simulink model "W15_test_scenario_Map_cs"  (R2019a)
settings: Solver=FixedStepDiscrete  StartTime=0.0  StopTime=40  FixedStep=1/20  RelTol=1e-3
PreLoadFcn:
  | mbxruntime.callbacks.PreLoadFcn(bdroot);
  | check_NUTS_defined
  | model_closed = 0;
  | assignin('base',['model_closed_' bdroot],false);
PostLoadFcn:
  | mbxruntime.callbacks.PostLoadFcn(bdroot);
InitFcn:
  | mbxruntime.callbacks.InitFcn(bdroot);
StartFcn:
  | mbxruntime.callbacks.StartFcn(bdroot);
StopFcn:
  | mbxruntime.callbacks.StopFcn(bdroot);;
  | 
model workspace: external: MAT-File .\W15_test_scenario_Map_cs_hws.mat (data not in the file)
undefined symbols (not defined in the file or in its folder): DiscIntNeverNeededParam, Header, InitImageOutputDir, mbxruntime, Orientation, Poses, Poses_SL_Info, Position, tabledata, W15_test_scenario_Map_cs_169a523538b1c731, W15_test_scenario_Map_cs_214b7e80d33618ad, W15_test_scenario_Map_cs_2206180be8b5ba9f, W15_test_scenario_Map_cs_268dfee03830d0a5, W15_test_scenario_Map_cs_347647b3d0c1b5a3, W15_test_scenario_Map_cs_358fdd58312a0833, W15_test_scenario_Map_cs_5ba16ded7c4f6682, W15_test_scenario_Map_cs_615f57972979d30a, W15_test_scenario_Map_cs_62d25263d5c47c08, W15_test_scenario_Map_cs_6d9a3b1c984f4232, W15_test_scenario_Map_cs_8e30bed0320ac6d2, W15_test_scenario_Map_cs_91166841717f8002, W15_test_scenario_Map_cs_ab37b8bb7c840172, W15_test_scenario_Map_cs_Audi_A8_Sedan_1_Path_pathUniqueID, W15_test_scenario_Map_cs_bc72e7b61fa128bc, W15_test_scenario_Map_cs_Child_RegularAni_1_Path_pathUniqueID, W15_test_scenario_Map_cs_Child_RegularAni_2_Path_pathUniqueID, W15_test_scenario_Map_cs_e2220a37b0e8fe8c, W15_test_scenario_Map_cs_e86a0965b14e60bb, W15_test_scenario_Map_cs_Female_RegularAni_1_Path_pathUniqueID, W15_test_scenario_Map_cs_Male_RegularAni_1_Path_pathUniqueID, W15_test_scenario_Map_cs_Male_RegularAni_2_Path_pathUniqueID
libraries: simulink_extras x30, adeye_lib x14, simulink x10, robotlib x4, sharedtransform x2, PreScanSimulinkLibrary x2, PreScanUsefulBlocks x1
(part 4 of 8)

== system W15_test_scenario_Map_cs/STATE_Audi_A8_Sedan_1_bus ==
  STATE_Audi_A8_Sedan_1_bus : Inport  Tag=inport/StatePort  OutDataTypeStr=Bus: PRESCAN_STATEACTUATORDATA  PortDimensions=1  SampleTime=1/20  BusOutputAsStruct=on
  Actuator : S-Function  FunctionName=sfun_StateActuator  Parameters=mbxruntime.parameters.convert(UniqueID), mbxruntime.parameters.convert(TimeStep)  SFunctionDeploymentMode=off  EnableBusSupport=off  mask(PreScan Sink Block: State){UniqueID=18645, TimeStep=1/20}
      mask prompts: UniqueID "Auto-Assigned: Unique ID"; TimeStep "Auto-Assigned: Upload Period [s]"
      mask help:
      | The Actor State contains a vector signal of size (9x1), containing the following signals:
      |
      | -  Position    	(x,y,z)             	[m]
      | -  Velocity    	(vx,vy,vz)         	[m/s]
      | -  Angles       	(Roll, Pitch, Yaw)	[rad]
      |
      | The Actor state is defined in the global axis system.
      | The state is superponed on the Initial position defined in the GUI.
      |
      | For more information, please click Help.
      mask Help: eval('openHelp(222)')
      mask Display: image(imread('State.png'))
  wires:
  STATE_Audi_A8_Sedan_1_bus/1 -> Actuator/1

== system W15_test_scenario_Map_cs/STATE_BMW_X5_SUV_1_bus ==
  STATE_BMW_X5_SUV_1_bus : Inport  Tag=inport/StatePort  OutDataTypeStr=Bus: PRESCAN_STATEACTUATORDATA  PortDimensions=1  SampleTime=1/20  BusOutputAsStruct=on
  Actuator : S-Function  FunctionName=sfun_StateActuator  Parameters=mbxruntime.parameters.convert(UniqueID), mbxruntime.parameters.convert(TimeStep)  SFunctionDeploymentMode=off  EnableBusSupport=off  mask(PreScan Sink Block: State){UniqueID=9040, TimeStep=1/20}
      mask prompts: UniqueID "Auto-Assigned: Unique ID"; TimeStep "Auto-Assigned: Upload Period [s]"
      mask help:
      | The Actor State contains a vector signal of size (9x1), containing the following signals:
      |
      | -  Position    	(x,y,z)             	[m]
      | -  Velocity    	(vx,vy,vz)         	[m/s]
      | -  Angles       	(Roll, Pitch, Yaw)	[rad]
      |
      | The Actor state is defined in the global axis system.
      | The state is superponed on the Initial position defined in the GUI.
      |
      | For more information, please click Help.
      mask Help: eval('openHelp(222)')
      mask Display: image(imread('State.png'))
  wires:
  STATE_BMW_X5_SUV_1_bus/1 -> Actuator/1

== system W15_test_scenario_Map_cs/STATE_Child_RegularAni_1_bus ==
  STATE_Child_RegularAni_1_bus : Inport  Tag=inport/StatePort  OutDataTypeStr=Bus: PRESCAN_STATEACTUATORDATA  PortDimensions=1  SampleTime=1/20  BusOutputAsStruct=on
  Actuator : S-Function  FunctionName=sfun_StateActuator  Parameters=mbxruntime.parameters.convert(UniqueID), mbxruntime.parameters.convert(TimeStep)  SFunctionDeploymentMode=off  EnableBusSupport=off  mask(PreScan Sink Block: State){UniqueID=18395, TimeStep=1/20}
      mask prompts: UniqueID "Auto-Assigned: Unique ID"; TimeStep "Auto-Assigned: Upload Period [s]"
      mask help:
      | The Actor State contains a vector signal of size (9x1), containing the following signals:
      |
      | -  Position    	(x,y,z)             	[m]
      | -  Velocity    	(vx,vy,vz)         	[m/s]
      | -  Angles       	(Roll, Pitch, Yaw)	[rad]
      |
      | The Actor state is defined in the global axis system.
      | The state is superponed on the Initial position defined in the GUI.
      |
      | For more information, please click Help.
      mask Help: eval('openHelp(222)')
      mask Display: image(imread('State.png'))
  wires:
  STATE_Child_RegularAni_1_bus/1 -> Actuator/1

== system W15_test_scenario_Map_cs/STATE_Child_RegularAni_2_bus ==
  STATE_Child_RegularAni_2_bus : Inport  Tag=inport/StatePort  OutDataTypeStr=Bus: PRESCAN_STATEACTUATORDATA  PortDimensions=1  SampleTime=1/20  BusOutputAsStruct=on
  Actuator : S-Function  FunctionName=sfun_StateActuator  Parameters=mbxruntime.parameters.convert(UniqueID), mbxruntime.parameters.convert(TimeStep)  SFunctionDeploymentMode=off  EnableBusSupport=off  mask(PreScan Sink Block: State){UniqueID=18628, TimeStep=1/20}
      mask prompts: UniqueID "Auto-Assigned: Unique ID"; TimeStep "Auto-Assigned: Upload Period [s]"
      mask help:
      | The Actor State contains a vector signal of size (9x1), containing the following signals:
      |
      | -  Position    	(x,y,z)             	[m]
      | -  Velocity    	(vx,vy,vz)         	[m/s]
      | -  Angles       	(Roll, Pitch, Yaw)	[rad]
      |
      | The Actor state is defined in the global axis system.
      | The state is superponed on the Initial position defined in the GUI.
      |
      | For more information, please click Help.
      mask Help: eval('openHelp(222)')
      mask Display: image(imread('State.png'))
  wires:
  STATE_Child_RegularAni_2_bus/1 -> Actuator/1

== system W15_test_scenario_Map_cs/STATE_Citroen_C3_Hatchback_1_bus ==
  STATE_Citroen_C3_Hatchback_1_bus : Inport  Tag=inport/StatePort  OutDataTypeStr=Bus: PRESCAN_STATEACTUATORDATA  PortDimensions=1  SampleTime=1/20  BusOutputAsStruct=on
  Actuator : S-Function  FunctionName=sfun_StateActuator  Parameters=mbxruntime.parameters.convert(UniqueID), mbxruntime.parameters.convert(TimeStep)  SFunctionDeploymentMode=off  EnableBusSupport=off  mask(PreScan Sink Block: State){UniqueID=18857, TimeStep=1/20}
      mask prompts: UniqueID "Auto-Assigned: Unique ID"; TimeStep "Auto-Assigned: Upload Period [s]"
      mask help:
      | The Actor State contains a vector signal of size (9x1), containing the following signals:
      |
      | -  Position    	(x,y,z)             	[m]
      | -  Velocity    	(vx,vy,vz)         	[m/s]
      | -  Angles       	(Roll, Pitch, Yaw)	[rad]
      |
      | The Actor state is defined in the global axis system.
      | The state is superponed on the Initial position defined in the GUI.
      |
      | For more information, please click Help.
      mask Help: eval('openHelp(222)')
      mask Display: image(imread('State.png'))
  wires:
  STATE_Citroen_C3_Hatchback_1_bus/1 -> Actuator/1

== system W15_test_scenario_Map_cs/STATE_Female_RegularAni_1_bus ==
  STATE_Female_RegularAni_1_bus : Inport  Tag=inport/StatePort  OutDataTypeStr=Bus: PRESCAN_STATEACTUATORDATA  PortDimensions=1  SampleTime=1/20  BusOutputAsStruct=on
  Actuator : S-Function  FunctionName=sfun_StateActuator  Parameters=mbxruntime.parameters.convert(UniqueID), mbxruntime.parameters.convert(TimeStep)  SFunctionDeploymentMode=off  EnableBusSupport=off  mask(PreScan Sink Block: State){UniqueID=18631, TimeStep=1/20}
      mask prompts: UniqueID "Auto-Assigned: Unique ID"; TimeStep "Auto-Assigned: Upload Period [s]"
      mask help:
      | The Actor State contains a vector signal of size (9x1), containing the following signals:
      |
      | -  Position    	(x,y,z)             	[m]
      | -  Velocity    	(vx,vy,vz)         	[m/s]
      | -  Angles       	(Roll, Pitch, Yaw)	[rad]
      |
      | The Actor state is defined in the global axis system.
      | The state is superponed on the Initial position defined in the GUI.
      |
      | For more information, please click Help.
      mask Help: eval('openHelp(222)')
      mask Display: image(imread('State.png'))
  wires:
  STATE_Female_RegularAni_1_bus/1 -> Actuator/1

== system W15_test_scenario_Map_cs/STATE_Ford_Fiesta_Hatchback_1_bus ==
  STATE_Ford_Fiesta_Hatchback_1_bus : Inport  Tag=inport/StatePort  OutDataTypeStr=Bus: PRESCAN_STATEACTUATORDATA  PortDimensions=1  SampleTime=1/20  BusOutputAsStruct=on
  Actuator : S-Function  FunctionName=sfun_StateActuator  Parameters=mbxruntime.parameters.convert(UniqueID), mbxruntime.parameters.convert(TimeStep)  SFunctionDeploymentMode=off  EnableBusSupport=off  mask(PreScan Sink Block: State){UniqueID=4876, TimeStep=1/20}
      mask prompts: UniqueID "Auto-Assigned: Unique ID"; TimeStep "Auto-Assigned: Upload Period [s]"
      mask help:
      | The Actor State contains a vector signal of size (9x1), containing the following signals:
      |
      | -  Position    	(x,y,z)             	[m]
      | -  Velocity    	(vx,vy,vz)         	[m/s]
      | -  Angles       	(Roll, Pitch, Yaw)	[rad]
      |
      | The Actor state is defined in the global axis system.
      | The state is superponed on the Initial position defined in the GUI.
      |
      | For more information, please click Help.
      mask Help: eval('openHelp(222)')
      mask Display: image(imread('State.png'))
  wires:
  STATE_Ford_Fiesta_Hatchback_1_bus/1 -> Actuator/1

== system W15_test_scenario_Map_cs/STATE_Male_RegularAni_1_bus ==
  STATE_Male_RegularAni_1_bus : Inport  Tag=inport/StatePort  OutDataTypeStr=Bus: PRESCAN_STATEACTUATORDATA  PortDimensions=1  SampleTime=1/20  BusOutputAsStruct=on
  Actuator : S-Function  FunctionName=sfun_StateActuator  Parameters=mbxruntime.parameters.convert(UniqueID), mbxruntime.parameters.convert(TimeStep)  SFunctionDeploymentMode=off  EnableBusSupport=off  mask(PreScan Sink Block: State){UniqueID=18634, TimeStep=1/20}
      mask prompts: UniqueID "Auto-Assigned: Unique ID"; TimeStep "Auto-Assigned: Upload Period [s]"
      mask help:
      | The Actor State contains a vector signal of size (9x1), containing the following signals:
      |
      | -  Position    	(x,y,z)             	[m]
      | -  Velocity    	(vx,vy,vz)         	[m/s]
      | -  Angles       	(Roll, Pitch, Yaw)	[rad]
      |
      | The Actor state is defined in the global axis system.
      | The state is superponed on the Initial position defined in the GUI.
      |
      | For more information, please click Help.
      mask Help: eval('openHelp(222)')
      mask Display: image(imread('State.png'))
  wires:
  STATE_Male_RegularAni_1_bus/1 -> Actuator/1

== system W15_test_scenario_Map_cs/STATE_Male_RegularAni_2_bus ==
  STATE_Male_RegularAni_2_bus : Inport  Tag=inport/StatePort  OutDataTypeStr=Bus: PRESCAN_STATEACTUATORDATA  PortDimensions=1  SampleTime=1/20  BusOutputAsStruct=on
  Actuator : S-Function  FunctionName=sfun_StateActuator  Parameters=mbxruntime.parameters.convert(UniqueID), mbxruntime.parameters.convert(TimeStep)  SFunctionDeploymentMode=off  EnableBusSupport=off  mask(PreScan Sink Block: State){UniqueID=18853, TimeStep=1/20}
      mask prompts: UniqueID "Auto-Assigned: Unique ID"; TimeStep "Auto-Assigned: Upload Period [s]"
      mask help:
      | The Actor State contains a vector signal of size (9x1), containing the following signals:
      |
      | -  Position    	(x,y,z)             	[m]
      | -  Velocity    	(vx,vy,vz)         	[m/s]
      | -  Angles       	(Roll, Pitch, Yaw)	[rad]
      |
      | The Actor state is defined in the global axis system.
      | The state is superponed on the Initial position defined in the GUI.
      |
      | For more information, please click Help.
      mask Help: eval('openHelp(222)')
      mask Display: image(imread('State.png'))
  wires:
  STATE_Male_RegularAni_2_bus/1 -> Actuator/1

== system W15_test_scenario_Map_cs/ScenarioEngine ==
  Clock : Clock
  sfun_ScenarioEngine : S-Function  FunctionName=sfun_ScenarioEngine  Parameters=TimeStep  SFunctionDeploymentMode=off  EnableBusSupport=off
  wires:
  Clock/1 -> sfun_ScenarioEngine/1

== system W15_test_scenario_Map_cs/Synchronizer ==
  Bus Selector1 : BusSelector  OutputSignals=FederateStopped
  Stop Simulation : Stop
  sfun_Synchronizer : S-Function  FunctionName=sfun_Synchronizer  Parameters=SampleTime  SFunctionDeploymentMode=off  EnableBusSupport=off  mask(Legacy Function){SFunctionSpec=void prescan_synchronizer_outputFcn(void ** work1, PRESCAN_SYNCHRONIZEDATA y1[1]), SampleTime=TimeStep, ShowSpec=on}
      mask prompts: SampleTime "Sample time (-1 for inherited):"; ShowSpec "Display function specification"
      mask help:
      | This block allows you to call the legacy functions specified by the following Legacy Code Tool definition:
      | def.SFunctionName = 'sfun_Synchronizer';
      | def.OutputFcnSpec = 'void prescan_synchronizer_outputFcn(void ** work1, PRESCAN_TIMESTAMPDATA u1[1], PRESCAN_SYNCHRONIZEDATA y1[1])';
      | def.StartFcnSpec = 'void prescan_synchronizer_startFcn(void ** work1)';
      | def.TerminateFcnSpec = 'void prescan_synchronizer_terminateFcn(void ** work1)';
      | def.HeaderFiles = {'prescan_synchronizer_data.h'};
      | def.HostLibFiles = {'sensorinterfaced.lib'};
      | def.IncPaths = {'src', 'C:\prescandev\vislibrary\vis\..\pimp\include\sensors\InterfaceRTW'};
      | def.SrcPaths = {'src'};
      | def.LibPaths = {'C:\\prescandev\\vislibrary_build\lib'};
      | def.SampleTime = 'parameterized';
      | def.Options.language = 'C';
      mask Help: <p>This block was generated automatically by the Legacy Code Tool. For detailed help on this tool, call<a href="matlab:legacy_code('help')"> legacy_code('help')</a>.</p>
      mask Callback ShowSpec:
      | if strcmp(get_param(gcbh, 'ShowSpec'), 'on')
      |   set_param(gcbh, 'MaskDisplay', sprintf('fprintf(''%s'');', get_param(gcbh, 'SFunctionSpec')));
      | else
      |   set_param(gcbh, 'MaskDisplay', sprintf('fprintf(''%s'');', get_param(gcbh, 'FunctionName')));
      | end
      mask Display: fprintf('void prescan_synchronizer_outputFcn(void ** work1, PRESCAN_SYNCHRONIZEDATA y1[1])');
  wires:
  sfun_Synchronizer/1 -> Bus Selector1/1
  Bus Selector1/1 -> Stop Simulation/1  "<FederateStopped>"

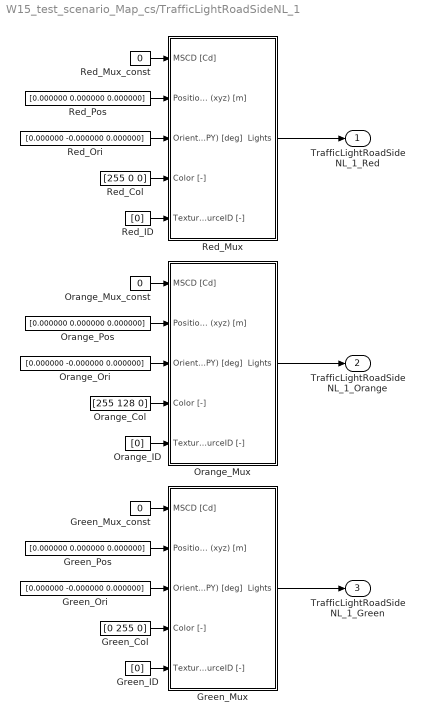
== system W15_test_scenario_Map_cs/TrafficLightRoadSideNL_1 ==
  Green_Col : Constant  Tag=VisuLightConst  Value=[0 255 0]
  Green_ID : Constant  Tag=VisuLightConst  Value=[0]
  Green_Mux : Subsystem  Tag=mux/ActiveLight  mask(PreScan User Interface: VisuActiveLight){}
      mask help:
      | The VisuActiveLight block provides a way for detailed animation of Light Sources, such as the indicator, brake, fog and main lights of a vehicle, or a light post.
      |
      | For more information, please click Help.
      settings: DeleteFcn=PreScanBlockDeleteFcn;
      mask Help: eval('openHelp(209)')
  Green_Mux_const : Constant  Tag=VisuLightConst  Value=0
  Green_Ori : Constant  Tag=VisuLightConst  Value=[0.000000 -0.000000 0.000000]
  Green_Pos : Constant  Tag=VisuLightConst  Value=[0.000000 0.000000 0.000000]
  Orange_Col : Constant  Tag=VisuLightConst  Value=[255 128 0]
  Orange_ID : Constant  Tag=VisuLightConst  Value=[0]
  Orange_Mux : Subsystem  Tag=mux/ActiveLight  mask(PreScan User Interface: VisuActiveLight){}
      mask help:
      | The VisuActiveLight block provides a way for detailed animation of Light Sources, such as the indicator, brake, fog and main lights of a vehicle, or a light post.
      |
      | For more information, please click Help.
      settings: DeleteFcn=PreScanBlockDeleteFcn;
      mask Help: eval('openHelp(209)')
  Orange_Mux_const : Constant  Tag=VisuLightConst  Value=0
  Orange_Ori : Constant  Tag=VisuLightConst  Value=[0.000000 -0.000000 0.000000]
  Orange_Pos : Constant  Tag=VisuLightConst  Value=[0.000000 0.000000 0.000000]
  Red_Col : Constant  Tag=VisuLightConst  Value=[255 0 0]
  Red_ID : Constant  Tag=VisuLightConst  Value=[0]
  Red_Mux : Subsystem  Tag=mux/ActiveLight  mask(PreScan User Interface: VisuActiveLight){}
      mask help:
      | The VisuActiveLight block provides a way for detailed animation of Light Sources, such as the indicator, brake, fog and main lights of a vehicle, or a light post.
      |
      | For more information, please click Help.
      settings: DeleteFcn=PreScanBlockDeleteFcn;
      mask Help: eval('openHelp(209)')
  Red_Mux_const : Constant  Tag=VisuLightConst  Value=0
  Red_Ori : Constant  Tag=VisuLightConst  Value=[0.000000 -0.000000 0.000000]
  Red_Pos : Constant  Tag=VisuLightConst  Value=[0.000000 0.000000 0.000000]
  TrafficLightRoadSideNL_1_Red : Outport  Tag=outport/Red  OutDataTypeStr=Bus: PRESCAN_VISULIGHTACTUATOR_DATA  SampleTime=1/20
  TrafficLightRoadSideNL_1_Orange : Outport  Tag=outport/Orange  Port=2  OutDataTypeStr=Bus: PRESCAN_VISULIGHTACTUATOR_DATA  SampleTime=1/20
  TrafficLightRoadSideNL_1_Green : Outport  Tag=outport/Green  Port=3  OutDataTypeStr=Bus: PRESCAN_VISULIGHTACTUATOR_DATA  SampleTime=1/20
  wires:
  Green_Mux_const/1 -> Green_Mux/1(MSCD [Cd])
  Orange_Mux_const/1 -> Orange_Mux/1(MSCD [Cd])
  Red_Mux_const/1 -> Red_Mux/1(MSCD [Cd])
  Red_Mux/1(Lights) -> TrafficLightRoadSideNL_1_Red/1
  Red_Pos/1 -> Red_Mux/2(Position (xyz) [m])
  Red_Ori/1 -> Red_Mux/3(Orientation (RPY) [deg])
  Red_Col/1 -> Red_Mux/4(Color [-])
  Red_ID/1 -> Red_Mux/5(TextureResourceID [-])
  Orange_Mux/1(Lights) -> TrafficLightRoadSideNL_1_Orange/1
  Orange_Pos/1 -> Orange_Mux/2(Position (xyz) [m])
  Orange_Ori/1 -> Orange_Mux/3(Orientation (RPY) [deg])
  Orange_Col/1 -> Orange_Mux/4(Color [-])
  Orange_ID/1 -> Orange_Mux/5(TextureResourceID [-])
  Green_Mux/1(Lights) -> TrafficLightRoadSideNL_1_Green/1
  Green_Pos/1 -> Green_Mux/2(Position (xyz) [m])
  Green_Ori/1 -> Green_Mux/3(Orientation (RPY) [deg])
  Green_Col/1 -> Green_Mux/4(Color [-])
  Green_ID/1 -> Green_Mux/5(TextureResourceID [-])

== system W15_test_scenario_Map_cs/TrafficLightRoadSideNL_1_Green ==
  TrafficLightRoadSideNL_1_Green : Inport  Tag=inport/Green  OutDataTypeStr=Bus: PRESCAN_VISULIGHTACTUATOR_DATA  SampleTime=1/20  BusOutputAsStruct=on
  Actuator : S-Function  FunctionName=sfun_VisuLightActuator  Parameters=mbxruntime.parameters.convert(UniqueID), mbxruntime.parameters.convert(LightName), mbxruntime.parameters.convert(PivotName), mbxruntime.parameters.convert(TextureResources), mbxruntime.parameters.convert(ColorsObjectName), mbxruntime.parameters.convert(MeshOnColor), mbxruntime.parameters.convert(MeshOffColor), tabledata, TimeStep  SFunctionDeploymentMode=off  EnableBusSupport=off  mask(PreScan Sink Block: VisuActiveLight){UniqueID=646, LightName=TrafficLightRoadSideNL_1.LightActuator_2_Green_ActiveLight, PivotName=TrafficLightRoadSideNL_1.Green, TextureResources={ 'Resources/LightMap/GeneralLight.png'}, ColorsObjectName=TrafficLightRoadSideNL_1.Green, MeshOnColor=[0  100    0  255    0  100    0  255  102  102  102  255    0  510    0  255], MeshOffColor=[0  100    0  255    0  100    0  255  102  102  102  255    0    0    0  255], TimeStep=1/20}
      mask prompts: UniqueID "Parent Unique Identifier"; LightName "Light"; PivotName "Pivot"; TextureResources "Texture Resources"; ColorsObjectName "Light Fixture Color Object"; MeshOnColor "Light Fixture On Color"; MeshOffColor "Light Fixture Off Color"; TimeStep "Simulink time step"
      mask help:
      | The VisuActiveLight block provides a way for detailed animation of Light Sources, such as the indicator, brake, fog and main lights of a vehicle, or a light post.
      |
      | For more information, please click Help.
      mask init:
      | [tabledata] = mbxruntime.parameters.table(UniqueID,LightName,PivotName,TextureResources,ColorsObjectName,MeshOnColor,MeshOffColor);
      mask Help: eval('openHelp(209)')
      mask Display: image(imread('HeadLight.png'))
  wires:
  TrafficLightRoadSideNL_1_Green/1 -> Actuator/1

== system W15_test_scenario_Map_cs/TrafficLightRoadSideNL_1_Orange ==
  TrafficLightRoadSideNL_1_Orange : Inport  Tag=inport/Orange  OutDataTypeStr=Bus: PRESCAN_VISULIGHTACTUATOR_DATA  SampleTime=1/20  BusOutputAsStruct=on
  Actuator : S-Function  FunctionName=sfun_VisuLightActuator  Parameters=mbxruntime.parameters.convert(UniqueID), mbxruntime.parameters.convert(LightName), mbxruntime.parameters.convert(PivotName), mbxruntime.parameters.convert(TextureResources), mbxruntime.parameters.convert(ColorsObjectName), mbxruntime.parameters.convert(MeshOnColor), mbxruntime.parameters.convert(MeshOffColor), tabledata, TimeStep  SFunctionDeploymentMode=off  EnableBusSupport=off  mask(PreScan Sink Block: VisuActiveLight){UniqueID=646, LightName=TrafficLightRoadSideNL_1.LightActuator_1_Orange_ActiveLight, PivotName=TrafficLightRoadSideNL_1.Orange, TextureResources={ 'Resources/LightMap/GeneralLight.png'}, ColorsObjectName=TrafficLightRoadSideNL_1.Orange, MeshOnColor=[100   50    0  255  100   50    0  255  102  102  102  255  510  256    0  255], MeshOffColor=[100   50    0  255  100   50    0  255  102  102  102  255    0    0    0  255], TimeStep=1/20}
      mask prompts: UniqueID "Parent Unique Identifier"; LightName "Light"; PivotName "Pivot"; TextureResources "Texture Resources"; ColorsObjectName "Light Fixture Color Object"; MeshOnColor "Light Fixture On Color"; MeshOffColor "Light Fixture Off Color"; TimeStep "Simulink time step"
      mask help:
      | The VisuActiveLight block provides a way for detailed animation of Light Sources, such as the indicator, brake, fog and main lights of a vehicle, or a light post.
      |
      | For more information, please click Help.
      mask init:
      | [tabledata] = mbxruntime.parameters.table(UniqueID,LightName,PivotName,TextureResources,ColorsObjectName,MeshOnColor,MeshOffColor);
      mask Help: eval('openHelp(209)')
      mask Display: image(imread('HeadLight.png'))
  wires:
  TrafficLightRoadSideNL_1_Orange/1 -> Actuator/1

== system W15_test_scenario_Map_cs/TrafficLightRoadSideNL_1_Red ==
  TrafficLightRoadSideNL_1_Red : Inport  Tag=inport/Red  OutDataTypeStr=Bus: PRESCAN_VISULIGHTACTUATOR_DATA  SampleTime=1/20  BusOutputAsStruct=on
  Actuator : S-Function  FunctionName=sfun_VisuLightActuator  Parameters=mbxruntime.parameters.convert(UniqueID), mbxruntime.parameters.convert(LightName), mbxruntime.parameters.convert(PivotName), mbxruntime.parameters.convert(TextureResources), mbxruntime.parameters.convert(ColorsObjectName), mbxruntime.parameters.convert(MeshOnColor), mbxruntime.parameters.convert(MeshOffColor), tabledata, TimeStep  SFunctionDeploymentMode=off  EnableBusSupport=off  mask(PreScan Sink Block: VisuActiveLight){UniqueID=646, LightName=TrafficLightRoadSideNL_1.LightActuator_0_Red_ActiveLight, PivotName=TrafficLightRoadSideNL_1.Red, TextureResources={ 'Resources/LightMap/GeneralLight.png'}, ColorsObjectName=TrafficLightRoadSideNL_1.Red, MeshOnColor=[100    0    0  255  100    0    0  255  102  102  102  255  510    0    0  255], MeshOffColor=[100    0    0  255  100    0    0  255  102  102  102  255    0    0    0  255], TimeStep=1/20}
      mask prompts: UniqueID "Parent Unique Identifier"; LightName "Light"; PivotName "Pivot"; TextureResources "Texture Resources"; ColorsObjectName "Light Fixture Color Object"; MeshOnColor "Light Fixture On Color"; MeshOffColor "Light Fixture Off Color"; TimeStep "Simulink time step"
      mask help:
      | The VisuActiveLight block provides a way for detailed animation of Light Sources, such as the indicator, brake, fog and main lights of a vehicle, or a light post.
      |
      | For more information, please click Help.
      mask init:
      | [tabledata] = mbxruntime.parameters.table(UniqueID,LightName,PivotName,TextureResources,ColorsObjectName,MeshOnColor,MeshOffColor);
      mask Help: eval('openHelp(209)')
      mask Display: image(imread('HeadLight.png'))
  wires:
  TrafficLightRoadSideNL_1_Red/1 -> Actuator/1

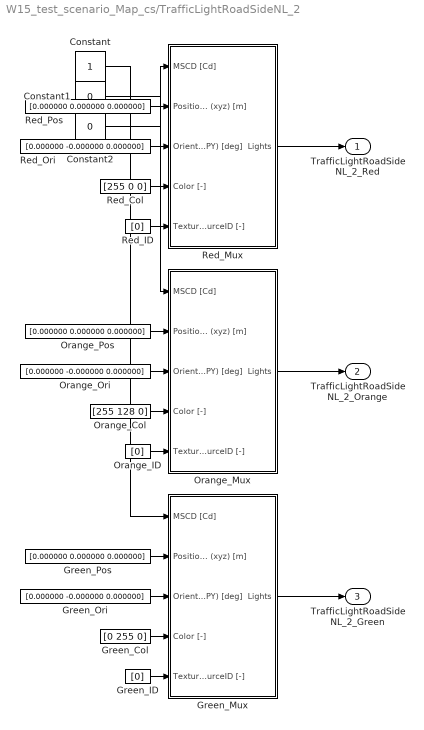
== system W15_test_scenario_Map_cs/TrafficLightRoadSideNL_2 ==
  Constant : Constant
  Constant1 : Constant  Value=0
  Constant2 : Constant  Value=0
  Green_Col : Constant  Tag=VisuLightConst  Value=[0 255 0]
  Green_ID : Constant  Tag=VisuLightConst  Value=[0]
  Green_Mux : Subsystem  Tag=mux/ActiveLight  mask(PreScan User Interface: VisuActiveLight){}
      mask help:
      | The VisuActiveLight block provides a way for detailed animation of Light Sources, such as the indicator, brake, fog and main lights of a vehicle, or a light post.
      |
      | For more information, please click Help.
      settings: DeleteFcn=PreScanBlockDeleteFcn;
      mask Help: eval('openHelp(209)')
  Green_Ori : Constant  Tag=VisuLightConst  Value=[0.000000 -0.000000 0.000000]
  Green_Pos : Constant  Tag=VisuLightConst  Value=[0.000000 0.000000 0.000000]
  Orange_Col : Constant  Tag=VisuLightConst  Value=[255 128 0]
  Orange_ID : Constant  Tag=VisuLightConst  Value=[0]
  Orange_Mux : Subsystem  Tag=mux/ActiveLight  mask(PreScan User Interface: VisuActiveLight){}
      mask help:
      | The VisuActiveLight block provides a way for detailed animation of Light Sources, such as the indicator, brake, fog and main lights of a vehicle, or a light post.
      |
      | For more information, please click Help.
      settings: DeleteFcn=PreScanBlockDeleteFcn;
      mask Help: eval('openHelp(209)')
  Orange_Ori : Constant  Tag=VisuLightConst  Value=[0.000000 -0.000000 0.000000]
  Orange_Pos : Constant  Tag=VisuLightConst  Value=[0.000000 0.000000 0.000000]
  Red_Col : Constant  Tag=VisuLightConst  Value=[255 0 0]
  Red_ID : Constant  Tag=VisuLightConst  Value=[0]
  Red_Mux : Subsystem  Tag=mux/ActiveLight  mask(PreScan User Interface: VisuActiveLight){}
      mask help:
      | The VisuActiveLight block provides a way for detailed animation of Light Sources, such as the indicator, brake, fog and main lights of a vehicle, or a light post.
      |
      | For more information, please click Help.
      settings: DeleteFcn=PreScanBlockDeleteFcn;
      mask Help: eval('openHelp(209)')
  Red_Ori : Constant  Tag=VisuLightConst  Value=[0.000000 -0.000000 0.000000]
  Red_Pos : Constant  Tag=VisuLightConst  Value=[0.000000 0.000000 0.000000]
  TrafficLightRoadSideNL_2_Red : Outport  Tag=outport/Red  OutDataTypeStr=Bus: PRESCAN_VISULIGHTACTUATOR_DATA  SampleTime=1/20
  TrafficLightRoadSideNL_2_Orange : Outport  Tag=outport/Orange  Port=2  OutDataTypeStr=Bus: PRESCAN_VISULIGHTACTUATOR_DATA  SampleTime=1/20
  TrafficLightRoadSideNL_2_Green : Outport  Tag=outport/Green  Port=3  OutDataTypeStr=Bus: PRESCAN_VISULIGHTACTUATOR_DATA  SampleTime=1/20
  wires:
  Constant/1 -> Green_Mux/1(MSCD [Cd])
  Constant1/1 -> Orange_Mux/1(MSCD [Cd])
  Constant2/1 -> Red_Mux/1(MSCD [Cd])
  Red_Mux/1(Lights) -> TrafficLightRoadSideNL_2_Red/1
  Red_Pos/1 -> Red_Mux/2(Position (xyz) [m])
  Red_Ori/1 -> Red_Mux/3(Orientation (RPY) [deg])
  Red_Col/1 -> Red_Mux/4(Color [-])
  Red_ID/1 -> Red_Mux/5(TextureResourceID [-])
  Orange_Mux/1(Lights) -> TrafficLightRoadSideNL_2_Orange/1
  Orange_Pos/1 -> Orange_Mux/2(Position (xyz) [m])
  Orange_Ori/1 -> Orange_Mux/3(Orientation (RPY) [deg])
  Orange_Col/1 -> Orange_Mux/4(Color [-])
  Orange_ID/1 -> Orange_Mux/5(TextureResourceID [-])
  Green_Mux/1(Lights) -> TrafficLightRoadSideNL_2_Green/1
  Green_Pos/1 -> Green_Mux/2(Position (xyz) [m])
  Green_Ori/1 -> Green_Mux/3(Orientation (RPY) [deg])
  Green_Col/1 -> Green_Mux/4(Color [-])
  Green_ID/1 -> Green_Mux/5(TextureResourceID [-])

== system W15_test_scenario_Map_cs/TrafficLightRoadSideNL_2_Green ==
  TrafficLightRoadSideNL_2_Green : Inport  Tag=inport/Green  OutDataTypeStr=Bus: PRESCAN_VISULIGHTACTUATOR_DATA  SampleTime=1/20  BusOutputAsStruct=on
  Actuator : S-Function  FunctionName=sfun_VisuLightActuator  Parameters=mbxruntime.parameters.convert(UniqueID), mbxruntime.parameters.convert(LightName), mbxruntime.parameters.convert(PivotName), mbxruntime.parameters.convert(TextureResources), mbxruntime.parameters.convert(ColorsObjectName), mbxruntime.parameters.convert(MeshOnColor), mbxruntime.parameters.convert(MeshOffColor), tabledata, TimeStep  SFunctionDeploymentMode=off  EnableBusSupport=off  mask(PreScan Sink Block: VisuActiveLight){UniqueID=647, LightName=TrafficLightRoadSideNL_2.LightActuator_2_Green_ActiveLight, PivotName=TrafficLightRoadSideNL_2.Green, TextureResources={ 'Resources/LightMap/GeneralLight.png'}, ColorsObjectName=TrafficLightRoadSideNL_2.Green, MeshOnColor=[0  100    0  255    0  100    0  255  102  102  102  255    0  510    0  255], MeshOffColor=[0  100    0  255    0  100    0  255  102  102  102  255    0    0    0  255], TimeStep=1/20}
      mask prompts: UniqueID "Parent Unique Identifier"; LightName "Light"; PivotName "Pivot"; TextureResources "Texture Resources"; ColorsObjectName "Light Fixture Color Object"; MeshOnColor "Light Fixture On Color"; MeshOffColor "Light Fixture Off Color"; TimeStep "Simulink time step"
      mask help:
      | The VisuActiveLight block provides a way for detailed animation of Light Sources, such as the indicator, brake, fog and main lights of a vehicle, or a light post.
      |
      | For more information, please click Help.
      mask init:
      | [tabledata] = mbxruntime.parameters.table(UniqueID,LightName,PivotName,TextureResources,ColorsObjectName,MeshOnColor,MeshOffColor);
      mask Help: eval('openHelp(209)')
      mask Display: image(imread('HeadLight.png'))
  wires:
  TrafficLightRoadSideNL_2_Green/1 -> Actuator/1

== system W15_test_scenario_Map_cs/TrafficLightRoadSideNL_2_Orange ==
  TrafficLightRoadSideNL_2_Orange : Inport  Tag=inport/Orange  OutDataTypeStr=Bus: PRESCAN_VISULIGHTACTUATOR_DATA  SampleTime=1/20  BusOutputAsStruct=on
  Actuator : S-Function  FunctionName=sfun_VisuLightActuator  Parameters=mbxruntime.parameters.convert(UniqueID), mbxruntime.parameters.convert(LightName), mbxruntime.parameters.convert(PivotName), mbxruntime.parameters.convert(TextureResources), mbxruntime.parameters.convert(ColorsObjectName), mbxruntime.parameters.convert(MeshOnColor), mbxruntime.parameters.convert(MeshOffColor), tabledata, TimeStep  SFunctionDeploymentMode=off  EnableBusSupport=off  mask(PreScan Sink Block: VisuActiveLight){UniqueID=647, LightName=TrafficLightRoadSideNL_2.LightActuator_1_Orange_ActiveLight, PivotName=TrafficLightRoadSideNL_2.Orange, TextureResources={ 'Resources/LightMap/GeneralLight.png'}, ColorsObjectName=TrafficLightRoadSideNL_2.Orange, MeshOnColor=[100   50    0  255  100   50    0  255  102  102  102  255  510  256    0  255], MeshOffColor=[100   50    0  255  100   50    0  255  102  102  102  255    0    0    0  255], TimeStep=1/20}
      mask prompts: UniqueID "Parent Unique Identifier"; LightName "Light"; PivotName "Pivot"; TextureResources "Texture Resources"; ColorsObjectName "Light Fixture Color Object"; MeshOnColor "Light Fixture On Color"; MeshOffColor "Light Fixture Off Color"; TimeStep "Simulink time step"
      mask help:
      | The VisuActiveLight block provides a way for detailed animation of Light Sources, such as the indicator, brake, fog and main lights of a vehicle, or a light post.
      |
      | For more information, please click Help.
      mask init:
      | [tabledata] = mbxruntime.parameters.table(UniqueID,LightName,PivotName,TextureResources,ColorsObjectName,MeshOnColor,MeshOffColor);
      mask Help: eval('openHelp(209)')
      mask Display: image(imread('HeadLight.png'))
  wires:
  TrafficLightRoadSideNL_2_Orange/1 -> Actuator/1

== system W15_test_scenario_Map_cs/TrafficLightRoadSideNL_2_Red ==
  TrafficLightRoadSideNL_2_Red : Inport  Tag=inport/Red  OutDataTypeStr=Bus: PRESCAN_VISULIGHTACTUATOR_DATA  SampleTime=1/20  BusOutputAsStruct=on
  Actuator : S-Function  FunctionName=sfun_VisuLightActuator  Parameters=mbxruntime.parameters.convert(UniqueID), mbxruntime.parameters.convert(LightName), mbxruntime.parameters.convert(PivotName), mbxruntime.parameters.convert(TextureResources), mbxruntime.parameters.convert(ColorsObjectName), mbxruntime.parameters.convert(MeshOnColor), mbxruntime.parameters.convert(MeshOffColor), tabledata, TimeStep  SFunctionDeploymentMode=off  EnableBusSupport=off  mask(PreScan Sink Block: VisuActiveLight){UniqueID=647, LightName=TrafficLightRoadSideNL_2.LightActuator_0_Red_ActiveLight, PivotName=TrafficLightRoadSideNL_2.Red, TextureResources={ 'Resources/LightMap/GeneralLight.png'}, ColorsObjectName=TrafficLightRoadSideNL_2.Red, MeshOnColor=[100    0    0  255  100    0    0  255  102  102  102  255  510    0    0  255], MeshOffColor=[100    0    0  255  100    0    0  255  102  102  102  255    0    0    0  255], TimeStep=1/20}
      mask prompts: UniqueID "Parent Unique Identifier"; LightName "Light"; PivotName "Pivot"; TextureResources "Texture Resources"; ColorsObjectName "Light Fixture Color Object"; MeshOnColor "Light Fixture On Color"; MeshOffColor "Light Fixture Off Color"; TimeStep "Simulink time step"
      mask help:
      | The VisuActiveLight block provides a way for detailed animation of Light Sources, such as the indicator, brake, fog and main lights of a vehicle, or a light post.
      |
      | For more information, please click Help.
      mask init:
      | [tabledata] = mbxruntime.parameters.table(UniqueID,LightName,PivotName,TextureResources,ColorsObjectName,MeshOnColor,MeshOffColor);
      mask Help: eval('openHelp(209)')
      mask Display: image(imread('HeadLight.png'))
  wires:
  TrafficLightRoadSideNL_2_Red/1 -> Actuator/1

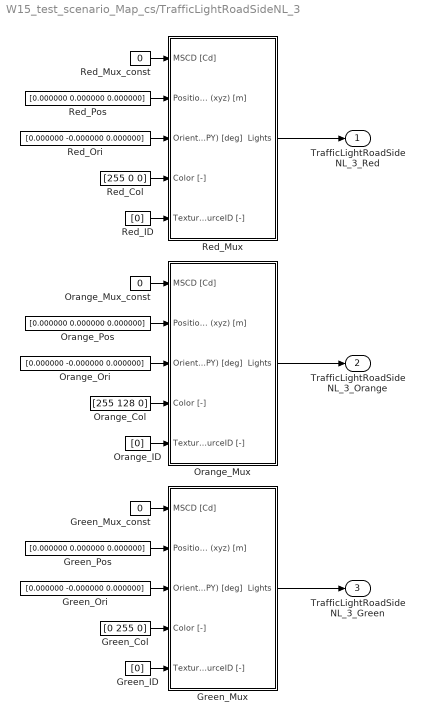
== system W15_test_scenario_Map_cs/TrafficLightRoadSideNL_3 ==
  Green_Col : Constant  Tag=VisuLightConst  Value=[0 255 0]
  Green_ID : Constant  Tag=VisuLightConst  Value=[0]
  Green_Mux : Subsystem  Tag=mux/ActiveLight  mask(PreScan User Interface: VisuActiveLight){}
      mask help:
      | The VisuActiveLight block provides a way for detailed animation of Light Sources, such as the indicator, brake, fog and main lights of a vehicle, or a light post.
      |
      | For more information, please click Help.
      settings: DeleteFcn=PreScanBlockDeleteFcn;
      mask Help: eval('openHelp(209)')
  Green_Mux_const : Constant  Tag=VisuLightConst  Value=0
  Green_Ori : Constant  Tag=VisuLightConst  Value=[0.000000 -0.000000 0.000000]
  Green_Pos : Constant  Tag=VisuLightConst  Value=[0.000000 0.000000 0.000000]
  Orange_Col : Constant  Tag=VisuLightConst  Value=[255 128 0]
  Orange_ID : Constant  Tag=VisuLightConst  Value=[0]
  Orange_Mux : Subsystem  Tag=mux/ActiveLight  mask(PreScan User Interface: VisuActiveLight){}
      mask help:
      | The VisuActiveLight block provides a way for detailed animation of Light Sources, such as the indicator, brake, fog and main lights of a vehicle, or a light post.
      |
      | For more information, please click Help.
      settings: DeleteFcn=PreScanBlockDeleteFcn;
      mask Help: eval('openHelp(209)')
  Orange_Mux_const : Constant  Tag=VisuLightConst  Value=0
  Orange_Ori : Constant  Tag=VisuLightConst  Value=[0.000000 -0.000000 0.000000]
  Orange_Pos : Constant  Tag=VisuLightConst  Value=[0.000000 0.000000 0.000000]
  Red_Col : Constant  Tag=VisuLightConst  Value=[255 0 0]
  Red_ID : Constant  Tag=VisuLightConst  Value=[0]
  Red_Mux : Subsystem  Tag=mux/ActiveLight  mask(PreScan User Interface: VisuActiveLight){}
      mask help:
      | The VisuActiveLight block provides a way for detailed animation of Light Sources, such as the indicator, brake, fog and main lights of a vehicle, or a light post.
      |
      | For more information, please click Help.
      settings: DeleteFcn=PreScanBlockDeleteFcn;
      mask Help: eval('openHelp(209)')
  Red_Mux_const : Constant  Tag=VisuLightConst  Value=0
  Red_Ori : Constant  Tag=VisuLightConst  Value=[0.000000 -0.000000 0.000000]
  Red_Pos : Constant  Tag=VisuLightConst  Value=[0.000000 0.000000 0.000000]
  TrafficLightRoadSideNL_3_Red : Outport  Tag=outport/Red  OutDataTypeStr=Bus: PRESCAN_VISULIGHTACTUATOR_DATA  SampleTime=1/20
  TrafficLightRoadSideNL_3_Orange : Outport  Tag=outport/Orange  Port=2  OutDataTypeStr=Bus: PRESCAN_VISULIGHTACTUATOR_DATA  SampleTime=1/20
  TrafficLightRoadSideNL_3_Green : Outport  Tag=outport/Green  Port=3  OutDataTypeStr=Bus: PRESCAN_VISULIGHTACTUATOR_DATA  SampleTime=1/20
  wires:
  Green_Mux_const/1 -> Green_Mux/1(MSCD [Cd])
  Orange_Mux_const/1 -> Orange_Mux/1(MSCD [Cd])
  Red_Mux_const/1 -> Red_Mux/1(MSCD [Cd])
  Red_Mux/1(Lights) -> TrafficLightRoadSideNL_3_Red/1
  Red_Pos/1 -> Red_Mux/2(Position (xyz) [m])
  Red_Ori/1 -> Red_Mux/3(Orientation (RPY) [deg])
  Red_Col/1 -> Red_Mux/4(Color [-])
  Red_ID/1 -> Red_Mux/5(TextureResourceID [-])
  Orange_Mux/1(Lights) -> TrafficLightRoadSideNL_3_Orange/1
  Orange_Pos/1 -> Orange_Mux/2(Position (xyz) [m])
  Orange_Ori/1 -> Orange_Mux/3(Orientation (RPY) [deg])
  Orange_Col/1 -> Orange_Mux/4(Color [-])
  Orange_ID/1 -> Orange_Mux/5(TextureResourceID [-])
  Green_Mux/1(Lights) -> TrafficLightRoadSideNL_3_Green/1
  Green_Pos/1 -> Green_Mux/2(Position (xyz) [m])
  Green_Ori/1 -> Green_Mux/3(Orientation (RPY) [deg])
  Green_Col/1 -> Green_Mux/4(Color [-])
  Green_ID/1 -> Green_Mux/5(TextureResourceID [-])

== system W15_test_scenario_Map_cs/TrafficLightRoadSideNL_3_Green ==
  TrafficLightRoadSideNL_3_Green : Inport  Tag=inport/Green  OutDataTypeStr=Bus: PRESCAN_VISULIGHTACTUATOR_DATA  SampleTime=1/20  BusOutputAsStruct=on
  Actuator : S-Function  FunctionName=sfun_VisuLightActuator  Parameters=mbxruntime.parameters.convert(UniqueID), mbxruntime.parameters.convert(LightName), mbxruntime.parameters.convert(PivotName), mbxruntime.parameters.convert(TextureResources), mbxruntime.parameters.convert(ColorsObjectName), mbxruntime.parameters.convert(MeshOnColor), mbxruntime.parameters.convert(MeshOffColor), tabledata, TimeStep  SFunctionDeploymentMode=off  EnableBusSupport=off  mask(PreScan Sink Block: VisuActiveLight){UniqueID=649, LightName=TrafficLightRoadSideNL_3.LightActuator_2_Green_ActiveLight, PivotName=TrafficLightRoadSideNL_3.Green, TextureResources={ 'Resources/LightMap/GeneralLight.png'}, ColorsObjectName=TrafficLightRoadSideNL_3.Green, MeshOnColor=[0  100    0  255    0  100    0  255  102  102  102  255    0  510    0  255], MeshOffColor=[0  100    0  255    0  100    0  255  102  102  102  255    0    0    0  255], TimeStep=1/20}
      mask prompts: UniqueID "Parent Unique Identifier"; LightName "Light"; PivotName "Pivot"; TextureResources "Texture Resources"; ColorsObjectName "Light Fixture Color Object"; MeshOnColor "Light Fixture On Color"; MeshOffColor "Light Fixture Off Color"; TimeStep "Simulink time step"
      mask help:
      | The VisuActiveLight block provides a way for detailed animation of Light Sources, such as the indicator, brake, fog and main lights of a vehicle, or a light post.
      |
      | For more information, please click Help.
      mask init:
      | [tabledata] = mbxruntime.parameters.table(UniqueID,LightName,PivotName,TextureResources,ColorsObjectName,MeshOnColor,MeshOffColor);
      mask Help: eval('openHelp(209)')
      mask Display: image(imread('HeadLight.png'))
  wires:
  TrafficLightRoadSideNL_3_Green/1 -> Actuator/1

== system W15_test_scenario_Map_cs/TrafficLightRoadSideNL_3_Orange ==
  TrafficLightRoadSideNL_3_Orange : Inport  Tag=inport/Orange  OutDataTypeStr=Bus: PRESCAN_VISULIGHTACTUATOR_DATA  SampleTime=1/20  BusOutputAsStruct=on
  Actuator : S-Function  FunctionName=sfun_VisuLightActuator  Parameters=mbxruntime.parameters.convert(UniqueID), mbxruntime.parameters.convert(LightName), mbxruntime.parameters.convert(PivotName), mbxruntime.parameters.convert(TextureResources), mbxruntime.parameters.convert(ColorsObjectName), mbxruntime.parameters.convert(MeshOnColor), mbxruntime.parameters.convert(MeshOffColor), tabledata, TimeStep  SFunctionDeploymentMode=off  EnableBusSupport=off  mask(PreScan Sink Block: VisuActiveLight){UniqueID=649, LightName=TrafficLightRoadSideNL_3.LightActuator_1_Orange_ActiveLight, PivotName=TrafficLightRoadSideNL_3.Orange, TextureResources={ 'Resources/LightMap/GeneralLight.png'}, ColorsObjectName=TrafficLightRoadSideNL_3.Orange, MeshOnColor=[100   50    0  255  100   50    0  255  102  102  102  255  510  256    0  255], MeshOffColor=[100   50    0  255  100   50    0  255  102  102  102  255    0    0    0  255], TimeStep=1/20}
      mask prompts: UniqueID "Parent Unique Identifier"; LightName "Light"; PivotName "Pivot"; TextureResources "Texture Resources"; ColorsObjectName "Light Fixture Color Object"; MeshOnColor "Light Fixture On Color"; MeshOffColor "Light Fixture Off Color"; TimeStep "Simulink time step"
      mask help:
      | The VisuActiveLight block provides a way for detailed animation of Light Sources, such as the indicator, brake, fog and main lights of a vehicle, or a light post.
      |
      | For more information, please click Help.
      mask init:
      | [tabledata] = mbxruntime.parameters.table(UniqueID,LightName,PivotName,TextureResources,ColorsObjectName,MeshOnColor,MeshOffColor);
      mask Help: eval('openHelp(209)')
      mask Display: image(imread('HeadLight.png'))
  wires:
  TrafficLightRoadSideNL_3_Orange/1 -> Actuator/1

== system W15_test_scenario_Map_cs/TrafficLightRoadSideNL_3_Red ==
  TrafficLightRoadSideNL_3_Red : Inport  Tag=inport/Red  OutDataTypeStr=Bus: PRESCAN_VISULIGHTACTUATOR_DATA  SampleTime=1/20  BusOutputAsStruct=on
  Actuator : S-Function  FunctionName=sfun_VisuLightActuator  Parameters=mbxruntime.parameters.convert(UniqueID), mbxruntime.parameters.convert(LightName), mbxruntime.parameters.convert(PivotName), mbxruntime.parameters.convert(TextureResources), mbxruntime.parameters.convert(ColorsObjectName), mbxruntime.parameters.convert(MeshOnColor), mbxruntime.parameters.convert(MeshOffColor), tabledata, TimeStep  SFunctionDeploymentMode=off  EnableBusSupport=off  mask(PreScan Sink Block: VisuActiveLight){UniqueID=649, LightName=TrafficLightRoadSideNL_3.LightActuator_0_Red_ActiveLight, PivotName=TrafficLightRoadSideNL_3.Red, TextureResources={ 'Resources/LightMap/GeneralLight.png'}, ColorsObjectName=TrafficLightRoadSideNL_3.Red, MeshOnColor=[100    0    0  255  100    0    0  255  102  102  102  255  510    0    0  255], MeshOffColor=[100    0    0  255  100    0    0  255  102  102  102  255    0    0    0  255], TimeStep=1/20}
      mask prompts: UniqueID "Parent Unique Identifier"; LightName "Light"; PivotName "Pivot"; TextureResources "Texture Resources"; ColorsObjectName "Light Fixture Color Object"; MeshOnColor "Light Fixture On Color"; MeshOffColor "Light Fixture Off Color"; TimeStep "Simulink time step"
      mask help:
      | The VisuActiveLight block provides a way for detailed animation of Light Sources, such as the indicator, brake, fog and main lights of a vehicle, or a light post.
      |
      | For more information, please click Help.
      mask init:
      | [tabledata] = mbxruntime.parameters.table(UniqueID,LightName,PivotName,TextureResources,ColorsObjectName,MeshOnColor,MeshOffColor);
      mask Help: eval('openHelp(209)')
      mask Display: image(imread('HeadLight.png'))
  wires:
  TrafficLightRoadSideNL_3_Red/1 -> Actuator/1

== system W15_test_scenario_Map_cs/TrafficLightRoadSideNL_4 ==
  Green_Col : Constant  Tag=VisuLightConst  Value=[0 255 0]
  Green_ID : Constant  Tag=VisuLightConst  Value=[0]
  Green_Mux : Subsystem  Tag=mux/ActiveLight  mask(PreScan User Interface: VisuActiveLight){}
      mask help:
      | The VisuActiveLight block provides a way for detailed animation of Light Sources, such as the indicator, brake, fog and main lights of a vehicle, or a light post.
      |
      | For more information, please click Help.
      settings: DeleteFcn=PreScanBlockDeleteFcn;
      mask Help: eval('openHelp(209)')
  Green_Mux_const : Constant  Tag=VisuLightConst  Value=0
  Green_Ori : Constant  Tag=VisuLightConst  Value=[0.000000 -0.000000 0.000000]
  Green_Pos : Constant  Tag=VisuLightConst  Value=[0.000000 0.000000 0.000000]
  Orange_Col : Constant  Tag=VisuLightConst  Value=[255 128 0]
  Orange_ID : Constant  Tag=VisuLightConst  Value=[0]
  Orange_Mux : Subsystem  Tag=mux/ActiveLight  mask(PreScan User Interface: VisuActiveLight){}
      mask help:
      | The VisuActiveLight block provides a way for detailed animation of Light Sources, such as the indicator, brake, fog and main lights of a vehicle, or a light post.
      |
      | For more information, please click Help.
      settings: DeleteFcn=PreScanBlockDeleteFcn;
      mask Help: eval('openHelp(209)')
  Orange_Mux_const : Constant  Tag=VisuLightConst  Value=0
  Orange_Ori : Constant  Tag=VisuLightConst  Value=[0.000000 -0.000000 0.000000]
  Orange_Pos : Constant  Tag=VisuLightConst  Value=[0.000000 0.000000 0.000000]
  Red_Col : Constant  Tag=VisuLightConst  Value=[255 0 0]
  Red_ID : Constant  Tag=VisuLightConst  Value=[0]
  Red_Mux : Subsystem  Tag=mux/ActiveLight  mask(PreScan User Interface: VisuActiveLight){}
      mask help:
      | The VisuActiveLight block provides a way for detailed animation of Light Sources, such as the indicator, brake, fog and main lights of a vehicle, or a light post.
      |
      | For more information, please click Help.
      settings: DeleteFcn=PreScanBlockDeleteFcn;
      mask Help: eval('openHelp(209)')
  Red_Mux_const : Constant  Tag=VisuLightConst  Value=0
  Red_Ori : Constant  Tag=VisuLightConst  Value=[0.000000 -0.000000 0.000000]
  Red_Pos : Constant  Tag=VisuLightConst  Value=[0.000000 0.000000 0.000000]
  TrafficLightRoadSideNL_4_Red : Outport  Tag=outport/Red  OutDataTypeStr=Bus: PRESCAN_VISULIGHTACTUATOR_DATA  SampleTime=1/20
  TrafficLightRoadSideNL_4_Orange : Outport  Tag=outport/Orange  Port=2  OutDataTypeStr=Bus: PRESCAN_VISULIGHTACTUATOR_DATA  SampleTime=1/20
  TrafficLightRoadSideNL_4_Green : Outport  Tag=outport/Green  Port=3  OutDataTypeStr=Bus: PRESCAN_VISULIGHTACTUATOR_DATA  SampleTime=1/20
  wires:
  Green_Mux_const/1 -> Green_Mux/1(MSCD [Cd])
  Orange_Mux_const/1 -> Orange_Mux/1(MSCD [Cd])
  Red_Mux_const/1 -> Red_Mux/1(MSCD [Cd])
  Red_Mux/1(Lights) -> TrafficLightRoadSideNL_4_Red/1
  Red_Pos/1 -> Red_Mux/2(Position (xyz) [m])
  Red_Ori/1 -> Red_Mux/3(Orientation (RPY) [deg])
  Red_Col/1 -> Red_Mux/4(Color [-])
  Red_ID/1 -> Red_Mux/5(TextureResourceID [-])
  Orange_Mux/1(Lights) -> TrafficLightRoadSideNL_4_Orange/1
  Orange_Pos/1 -> Orange_Mux/2(Position (xyz) [m])
  Orange_Ori/1 -> Orange_Mux/3(Orientation (RPY) [deg])
  Orange_Col/1 -> Orange_Mux/4(Color [-])
  Orange_ID/1 -> Orange_Mux/5(TextureResourceID [-])
  Green_Mux/1(Lights) -> TrafficLightRoadSideNL_4_Green/1
  Green_Pos/1 -> Green_Mux/2(Position (xyz) [m])
  Green_Ori/1 -> Green_Mux/3(Orientation (RPY) [deg])
  Green_Col/1 -> Green_Mux/4(Color [-])
  Green_ID/1 -> Green_Mux/5(TextureResourceID [-])

== system W15_test_scenario_Map_cs/TrafficLightRoadSideNL_4_Green ==
  TrafficLightRoadSideNL_4_Green : Inport  Tag=inport/Green  OutDataTypeStr=Bus: PRESCAN_VISULIGHTACTUATOR_DATA  SampleTime=1/20  BusOutputAsStruct=on
  Actuator : S-Function  FunctionName=sfun_VisuLightActuator  Parameters=mbxruntime.parameters.convert(UniqueID), mbxruntime.parameters.convert(LightName), mbxruntime.parameters.convert(PivotName), mbxruntime.parameters.convert(TextureResources), mbxruntime.parameters.convert(ColorsObjectName), mbxruntime.parameters.convert(MeshOnColor), mbxruntime.parameters.convert(MeshOffColor), tabledata, TimeStep  SFunctionDeploymentMode=off  EnableBusSupport=off  mask(PreScan Sink Block: VisuActiveLight){UniqueID=650, LightName=TrafficLightRoadSideNL_4.LightActuator_2_Green_ActiveLight, PivotName=TrafficLightRoadSideNL_4.Green, TextureResources={ 'Resources/LightMap/GeneralLight.png'}, ColorsObjectName=TrafficLightRoadSideNL_4.Green, MeshOnColor=[0  100    0  255    0  100    0  255  102  102  102  255    0  510    0  255], MeshOffColor=[0  100    0  255    0  100    0  255  102  102  102  255    0    0    0  255], TimeStep=1/20}
      mask prompts: UniqueID "Parent Unique Identifier"; LightName "Light"; PivotName "Pivot"; TextureResources "Texture Resources"; ColorsObjectName "Light Fixture Color Object"; MeshOnColor "Light Fixture On Color"; MeshOffColor "Light Fixture Off Color"; TimeStep "Simulink time step"
      mask help:
      | The VisuActiveLight block provides a way for detailed animation of Light Sources, such as the indicator, brake, fog and main lights of a vehicle, or a light post.
      |
      | For more information, please click Help.
      mask init:
      | [tabledata] = mbxruntime.parameters.table(UniqueID,LightName,PivotName,TextureResources,ColorsObjectName,MeshOnColor,MeshOffColor);
      mask Help: eval('openHelp(209)')
      mask Display: image(imread('HeadLight.png'))
  wires:
  TrafficLightRoadSideNL_4_Green/1 -> Actuator/1

== system W15_test_scenario_Map_cs/TrafficLightRoadSideNL_4_Orange ==
  TrafficLightRoadSideNL_4_Orange : Inport  Tag=inport/Orange  OutDataTypeStr=Bus: PRESCAN_VISULIGHTACTUATOR_DATA  SampleTime=1/20  BusOutputAsStruct=on
  Actuator : S-Function  FunctionName=sfun_VisuLightActuator  Parameters=mbxruntime.parameters.convert(UniqueID), mbxruntime.parameters.convert(LightName), mbxruntime.parameters.convert(PivotName), mbxruntime.parameters.convert(TextureResources), mbxruntime.parameters.convert(ColorsObjectName), mbxruntime.parameters.convert(MeshOnColor), mbxruntime.parameters.convert(MeshOffColor), tabledata, TimeStep  SFunctionDeploymentMode=off  EnableBusSupport=off  mask(PreScan Sink Block: VisuActiveLight){UniqueID=650, LightName=TrafficLightRoadSideNL_4.LightActuator_1_Orange_ActiveLight, PivotName=TrafficLightRoadSideNL_4.Orange, TextureResources={ 'Resources/LightMap/GeneralLight.png'}, ColorsObjectName=TrafficLightRoadSideNL_4.Orange, MeshOnColor=[100   50    0  255  100   50    0  255  102  102  102  255  510  256    0  255], MeshOffColor=[100   50    0  255  100   50    0  255  102  102  102  255    0    0    0  255], TimeStep=1/20}
      mask prompts: UniqueID "Parent Unique Identifier"; LightName "Light"; PivotName "Pivot"; TextureResources "Texture Resources"; ColorsObjectName "Light Fixture Color Object"; MeshOnColor "Light Fixture On Color"; MeshOffColor "Light Fixture Off Color"; TimeStep "Simulink time step"
      mask help:
      | The VisuActiveLight block provides a way for detailed animation of Light Sources, such as the indicator, brake, fog and main lights of a vehicle, or a light post.
      |
      | For more information, please click Help.
      mask init:
      | [tabledata] = mbxruntime.parameters.table(UniqueID,LightName,PivotName,TextureResources,ColorsObjectName,MeshOnColor,MeshOffColor);
      mask Help: eval('openHelp(209)')
      mask Display: image(imread('HeadLight.png'))
  wires:
  TrafficLightRoadSideNL_4_Orange/1 -> Actuator/1
